simulink model "EEE_Lab5_CSE21180"  (R2024b)
settings: Solver=VariableStepAuto  StartTime=0.0  StopTime=0.2  RelTol=1e-3
libraries: spsSeriesRLCBranchLib x10, spsACVoltageSourceLib x6, spsDiodeLib x6, spsVoltageMeasurementLib x6, sps_lib x1
settings Model: Creator=Karthik  LastModifiedBy=surmy

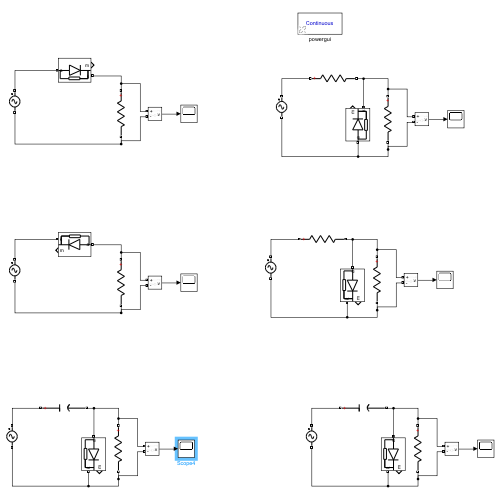
[thumbnail: Simulink's stored preview of the top-level diagram]
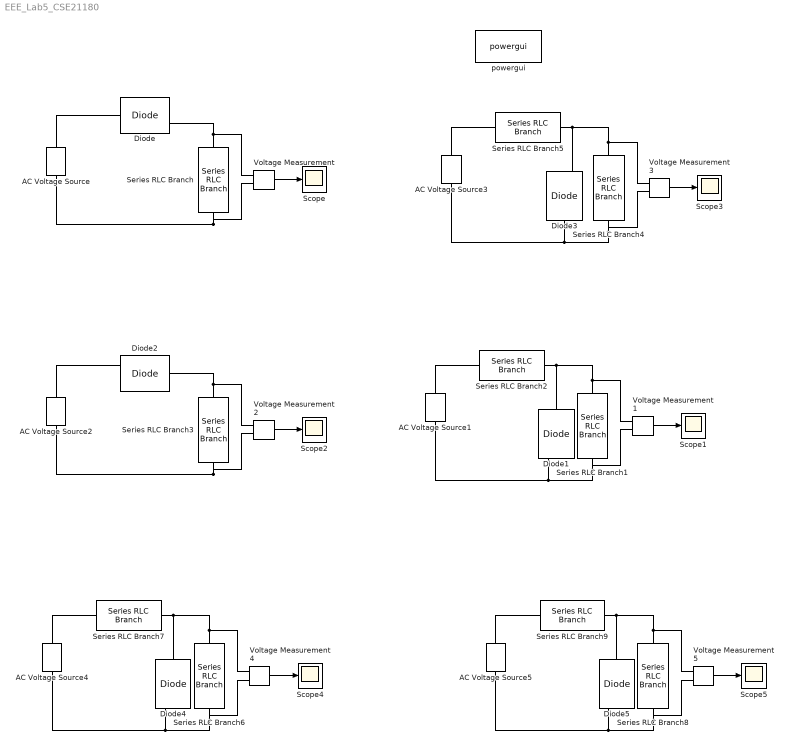
== system EEE_Lab5_CSE21180 ==
  AC Voltage Source{,1..5} (6 alike) : spsACVoltageSourceLib/AC Voltage Source  Amplitude=100  Phase=0  Frequency=60  SampleTime=0  Measurements=None  BusType=swing  Pref=10e3  Qref=0  Qmin=-inf  Qmax=+inf
  Diode{,1..5} (6 alike) : spsDiodeLib/Diode  Ron=0.001  Lon=0  Vf=0.8  IC=0  UseSnubber=0  Rs=500  Cs=250e-9  Measurements=on
  Scope{,1..5} (6 alike) : Scope
  Series RLC Branch{,1..6,8} (8 alike) : spsSeriesRLCBranchLib/Series RLC Branch  LConnTagsString=__new0  RConnTagsString=__new0  BranchType=R  Resistance=10  Inductance=1e-3  SetiL0=off  InitialCurrent=0  Capacitance=1e-6  Setx0=off  InitialVoltage=0  Measurements=None
  Series RLC Branch7 : spsSeriesRLCBranchLib/Series RLC Branch  LConnTagsString=__new0  RConnTagsString=__new0  BranchType=C  Resistance=10  Inductance=1e-3  SetiL0=off  InitialCurrent=0  Capacitance=1e-2  Setx0=off  InitialVoltage=0  Measurements=None
  Series RLC Branch9 : spsSeriesRLCBranchLib/Series RLC Branch  LConnTagsString=__new0  RConnTagsString=__new0  BranchType=C  Resistance=10  Inductance=1e-3  SetiL0=off  InitialCurrent=0  Capacitance=1e-2  Setx0=off  InitialVoltage=0  Measurements=None
  Voltage Measurement{,1..5} (6 alike) : spsVoltageMeasurementLib/Voltage Measurement  PhasorSimulation=off  OutputType=Complex  PSBequivalent=0
  powergui : sps_lib/powergui  Priority=1  SimulationMode=Continuous  SampleTime=50e-6  frequency=60  Iterations=50  frequencyindice=60  Pbase=100e6  ErrMax=1e-4  UnitsV=kV  UnitsW=MW  buscounter=0  FunctionMessages=off  echomessages=off  EnableUseOfTLC=off  CurrentSourceSwitches=off  DisableSnubberDevices=off  DisableRonSwitches=off  DisableVfSwitches=off  DisplayEquations=off  AutomaticDiscreteSolvers=off  SolverType=Tustin/Backward Euler (TBE)  Interpol=off  ExternalGateDelay=off  methode=off  Ts=100  x0status=blocks  SPID=on  SwTol=0  HookPort=off  NonlinearTolerance=1e-4  nMaxIteration=100  ContinueOnMaxIteration=off  RestoreLinks=warning  ResistiveCurrentMeasurement=off  Frange=[0:2:500]  Ylog=off  Xlog=on  ShowGrid=off  save=off  variable=ZData  structure=0  ZoomFFT=off  StartTime=0.0  cycles=1  DisplayStyle=1  fundamental=60  FreqAxis=off  MaxFrequency=1000  frequencyindicesteady=1  RmsSteady=1  display=off
  wires:
  Voltage Measurement/1 -> Scope/1
  Voltage Measurement2/1 -> Scope2/1
  Voltage Measurement3/1 -> Scope3/1
  Voltage Measurement4/1 -> Scope4/1
  Voltage Measurement5/1 -> Scope5/1
  Voltage Measurement1/1 -> Scope1/1
  connections:
  AC Voltage Source/RConn1 -- Diode/LConn1
  Series RLC Branch/LConn1 -- Voltage Measurement/LConn1 -- Diode/RConn1
  AC Voltage Source/LConn1 -- Voltage Measurement/LConn2 -- Series RLC Branch/RConn1
  AC Voltage Source2/LConn1 -- Voltage Measurement2/LConn2 -- Series RLC Branch3/RConn1
  Series RLC Branch4/LConn1 -- Diode3/RConn1 -- Series RLC Branch5/RConn1 -- Voltage Measurement3/LConn1
  Series RLC Branch4/RConn1 -- Diode3/LConn1 -- AC Voltage Source3/LConn1 -- Voltage Measurement3/LConn2
  Series RLC Branch3/LConn1 -- Diode2/LConn1 -- Voltage Measurement2/LConn1
  Diode2/RConn1 -- AC Voltage Source2/RConn1
  AC Voltage Source3/RConn1 -- Series RLC Branch5/LConn1
  Series RLC Branch6/LConn1 -- Diode4/LConn1 -- Series RLC Branch7/RConn1 -- Voltage Measurement4/LConn1
  Series RLC Branch6/RConn1 -- Diode4/RConn1 -- AC Voltage Source4/LConn1 -- Voltage Measurement4/LConn2
  AC Voltage Source4/RConn1 -- Series RLC Branch7/LConn1
  Series RLC Branch8/LConn1 -- Diode5/LConn1 -- Series RLC Branch9/RConn1 -- Voltage Measurement5/LConn1
  Series RLC Branch8/RConn1 -- Diode5/RConn1 -- AC Voltage Source5/LConn1 -- Voltage Measurement5/LConn2
  AC Voltage Source5/RConn1 -- Series RLC Branch9/LConn1
  Series RLC Branch1/RConn1 -- AC Voltage Source1/LConn1 -- Diode1/RConn1 -- Voltage Measurement1/LConn2
  Voltage Measurement1/LConn1 -- Series RLC Branch1/LConn1 -- Diode1/LConn1 -- Series RLC Branch2/RConn1
  AC Voltage Source1/RConn1 -- Series RLC Branch2/LConn1
